simulink model "obs_servo_full"  (R2022a)
settings: Solver=VariableStepAuto  StartTime=0.0  StopTime=20  RelTol=1e-3
values from neighbouring files (symbols this model uses):
  A = [0 0 0 1 0 0 ... (first row only)    [main.m]
  B = [0 0 ... (first row only)    [main.m]
  C = [1 0 0 0 0 0 ... (first row only)    [main.m]
  ka53 = real(inv(R)*Ba53'*P2)    [main.m]
  L = koo'    [main.m]
  ysp = -0.1*C*inv(A)*B*[-0.5+(a-b)/20;0.1+(b-c/(a+d+10))]    [main.m]
settings Model: Creator=wyton  LastModifiedBy=dzsgy
settings SolverCC: AlgebraicLoopSolver=TrustRegion
settings DebuggingCC: UnconnectedInputMsg=warning  UnconnectedOutputMsg=warning  UnconnectedLineMsg=warning  SFMachineParentedDataDiag=warning

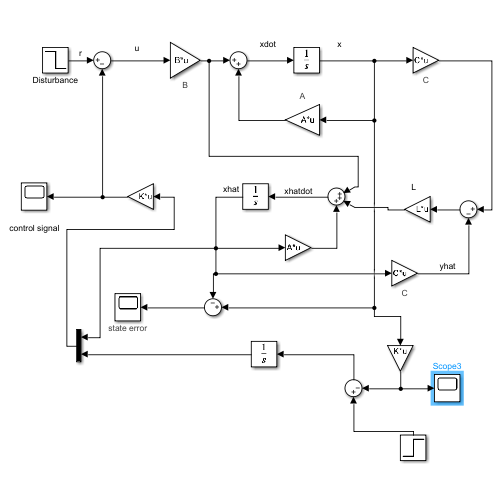
[thumbnail: Simulink's stored preview of the top-level diagram]
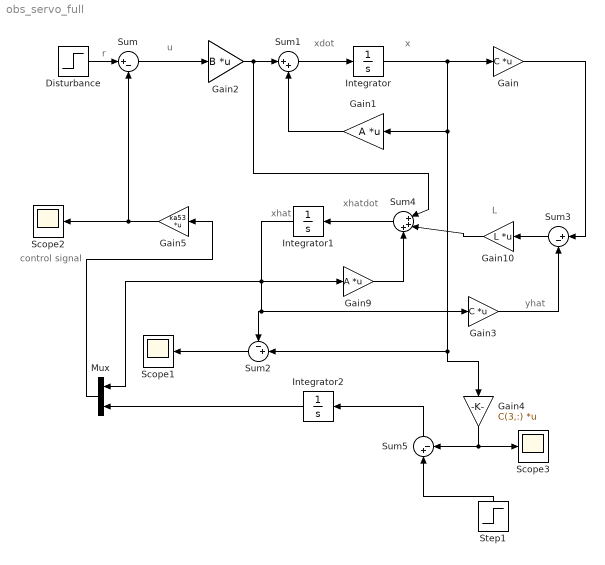
== system obs_servo_full ==
  note: u
  note: xhatdot
  note: x
  note: xdot
  note: yhat
  note: xhat
  note: control signal
  note: r
  note: L
  Disturbance : Step  Time=10  After=[-1,1]  SampleTime=0
  Gain : Gain  Gain=C  Multiplication=Matrix(K*u)
      settings: AttributesFormatString=C
  Gain1 : Gain  Gain=A  Multiplication=Matrix(K*u)
      settings: AttributesFormatString=A
  Gain10 : Gain  Gain=L  Multiplication=Matrix(K*u)
  Gain2 : Gain  Tag=B  Gain=B  Multiplication=Matrix(K*u)
      settings: AttributesFormatString=B
  Gain3 : Gain  Gain=C  Multiplication=Matrix(K*u)
      settings: AttributesFormatString=C
  Gain4 : Gain  Gain=C(3,:)  Multiplication=Matrix(K*u)
  Gain5 : Gain  Gain=ka53  Multiplication=Matrix(K*u)
  Gain9 : Gain  Gain=A  Multiplication=Matrix(K*u)
  Integrator : Integrator
  Integrator1 : Integrator
  Integrator2 : Integrator
  Mux : Mux  Inputs=2
  Scope1 : Scope
      settings: AttributesFormatString=state error
  Scope2 : Scope
  Scope3 : Scope
  Step1 : Step  Time=0  After=ysp(3)  SampleTime=0
  Sum : Sum  Inputs=|+-
  Sum1 : Sum  Inputs=|++
  Sum2 : Sum  Inputs=-+|
  Sum3 : Sum  Inputs=|+-
  Sum4 : Sum  Inputs=|+++
  Sum5 : Sum  Inputs=|+-
  wires:
  Disturbance/1 -> Sum/1
  Sum/1 -> Gain2/1
  Sum1/1 -> Integrator/1
  Integrator/1 -> Gain4/1, Sum2/2, Gain1/1, Gain/1
  Gain1/1 -> Sum1/2
  Gain5/1 -> Sum/2, Scope2/1
  Sum4/1 -> Integrator1/1
  Gain9/1 -> Sum4/3
  Gain10/1 -> Sum4/2
  Gain2/1 -> Sum4/1, Sum1/1
  Sum2/1 -> Scope1/1
  Sum3/1 -> Gain10/1
  Gain3/1 -> Sum3/2
  Integrator1/1 -> Mux/1, Gain3/1, Sum2/1, Gain9/1
  Step1/1 -> Sum5/1
  Integrator2/1 -> Mux/2
  Gain/1 -> Sum3/1
  Sum5/1 -> Integrator2/1
  Mux/1 -> Gain5/1
  Gain4/1 -> Scope3/1, Sum5/2
